simulink model "test_8m_0508"  (R2024a)
settings: Solver=FixedStepAuto  StartTime=0.0  StopTime=30  FixedStep=dt  RelTol=1e-3
values from neighbouring files (symbols this model uses):
  attitude_0 = [0; -90;  -0]    [ini_param_8m_0522.m]
  b = 4.0    (= 4)    [ini_param_8m_0522.m]
  cbar = 0.75    [ini_param_8m_0522.m]
  dt = 0.004    [ini_param_8m_0522.m]
  H = 1000    [ini_param_8m_0522.m]
  N_data = [0,200, 491, 804, 1077, 1344, 1559, 1832, 2078, 2318, 2579,            2864, 3117, 3371, 3608.2, 3872, 4055.7, 4291, 4507, 4739, 4935]'    [cal_motor.m]
  N_pwm = 0.01*[0, 5 ,10 ,15 ,20 ,25 ,30 ,35,40, 45 ,50 ,              55 ,60 ,65 ,70, 75, 80 , 85 ,90 ,95 ,100]'    [cal_motor.m]
  pitch_rate_K = 1    [ini_param_8m_0522.m]
  roll_rate_K = 1    [ini_param_8m_0522.m]
  S = 6.0    (= 6)    [ini_param_8m_0522.m]
  Ts = 0.05    [ini_param_8m_0522.m]
  Ts_sur = 0.25    [ini_param_8m_0522.m]
  yaw_rate_K = 1    [ini_param_8m_0522.m]
undefined symbols (not defined in the file or in its folder): sigbuilder_block, UAV
libraries: slpidlib x9, simulink_extras x6, sharedtransform x2, shared6dof x1
(part 1 of 11)
settings Model: Creator=elecl  LastModifiedBy=elecl

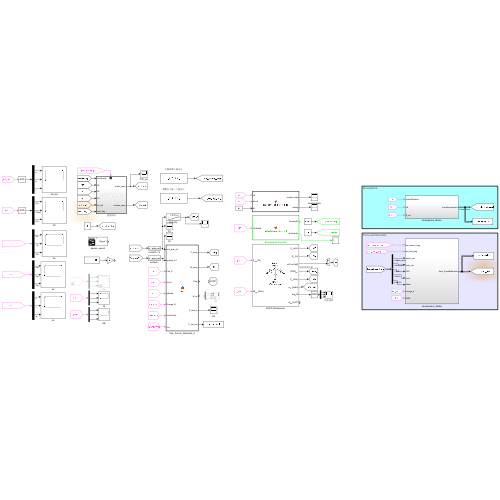
[thumbnail: Simulink's stored preview of the top-level diagram]
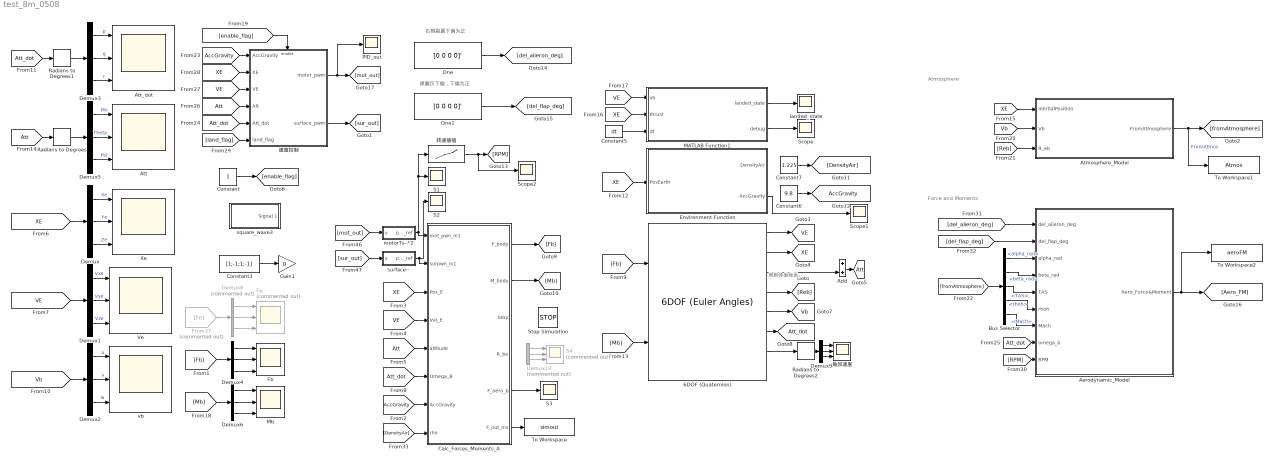
== system test_8m_0508 ==
  note: 地到体坐标系
  note: Force and Moments
  note: Atmosphere
  note: 右侧副翼下偏为正
  note: 襟翼仅下偏，下偏为正
  6DOF (Quaternion) : shared6dof/6DOF (Euler Angles)  units=Metric (MKS)  mtype=Fixed  rep=Quaternion  xme_0=[0 0 -H]  Vm_0=[1e-8 0 0]  eul_0=attitude_0*pi/180  pm_0=[0 0 0]  mass_0=StructAircraft.m  mass_e=0.5  mass_f=2.0  inertia=StructAircraft.inertia  inertia_e=eye(3)  inertia_f=2*eye(3)  k_quat=1.0  vre_flag=on  abi_flag=off  aMode=0  xme_statename=''  Vm_statename=''  eul_statename=''  quat_statename=''  pm_statename=''  mass_statename=''
  Add : Sum
  Aerodynamic_Model : Subsystem
  Atmosphere_Model : Subsystem
  Att : Scope  NumInputPorts=3
  Att_dot : Scope  NumInputPorts=3
  Bus Selector : BusSelector  OutputSignals=alpha_rad,beta_rad,TAS,rhoh,Mach
  Calc_Forces_Moments_A : MATLAB Function  TreatAsAtomicUnit=on  SystemSampleTime=0.004
  Constant : Constant
  Constant3 : Constant  Value=[1;-1;1;-1]
  Constant5 : Constant  Value=dt
  Constant6 : Constant  Value=9.8
  Constant7 : Constant  Value=1.225
  Demux{,1..6,9} (8 alike) : Demux  Outputs=3
  Demux10 : Demux  Commented=on  Outputs=3
  Demux8 : Demux  Commented=on  Outputs=3
  Environment Function : MATLAB Function  TreatAsAtomicUnit=on
  Fb : Scope  NumInputPorts=3
  Fe : Scope  Commented=on  NumInputPorts=3
  From37 : From  Commented=on  GotoTag=Fe
  Gain1 : Gain  Gain=0
  MATLAB Function1 : MATLAB Function  TreatAsAtomicUnit=on  SystemSampleTime=dt
  Mb : Scope  NumInputPorts=3
  One : Constant  Value=[0 0 0 0]'  OutDataTypeStr=Inherit: Inherit via back propagation
  One1 : Constant  Value=[0 0 0 0]'  OutDataTypeStr=Inherit: Inherit via back propagation
  PID_out : Scope
  Radians to Degrees : simulink_extras/Transformations/Radians to Degrees
  Radians to Degrees1 : simulink_extras/Transformations/Radians to Degrees
  Radians to Degrees2 : simulink_extras/Transformations/Radians to Degrees
  S1 : Scope
  S2 : Scope
  S3 : Scope
  S4 : Scope  Commented=on  NumInputPorts=3
  Scope : Scope
  Scope1 : Scope
  Scope2 : Scope
  Stop Simulation : Stop
  To Workspace : ToWorkspace  VariableName=simout  SaveFormat=Structure With Time  SampleTime=1
  To Workspace1 : ToWorkspace  VariableName=Atmos  SaveFormat=Structure  SampleTime=0.02
  To Workspace2 : ToWorkspace  VariableName=aeroFM  SaveFormat=Structure  SampleTime=0.02
  Ve : Scope  NumInputPorts=3
  Xe : Scope  NumInputPorts=3
  landed_state : Scope
  motorTs--*2 : Subsystem
  square_wave3 : Subsystem  Tag=STV Subsys  LoadFcn=sigbuilder_block('load');  StartFcn=sigbuilder_block('start');  StopFcn=sigbuilder_block('stop');  ClipboardFcn=sigbuilder_block('clipboard');  mask(Sigbuilder block){tuvar=[0:10]}
      mask help: Simulink:masks:SigbuilderBlock_MD
      mask init:
      | if ~strcmp(get_param(bdroot(gcbh),'SimulationStatus'),'stopped') tuvar = sigbuilder_block('maskInit'); end
      settings: CopyFcn=sigbuilder_block('copy');  DeleteFcn=sigbuilder_block('delete');  ModelCloseFcn=sigbuilder_block('modelClose');  PreSaveFcn=sigbuilder_block('preSave');  PauseFcn=sigbuilder_block('pause');  ContinueFcn=sigbuilder_block('continue');  NameChangeFcn=sigbuilder_block('namechange');  OpenFcn=sigbuilder_block('open',[239.25 91.5 550.5 408.75 ]);  CloseFcn=sigbuilder_block('close');
      mask Display: plot(0, 0, 100, 100,[2, 2, 32, 32, 2], [68, 8, 8, 68, 68],[32, 2], [38, 38], [32, 19, 2],[53, 60, 44], [32, 17, 17, 2],[16, 16, 31, 31]);txt = getActiveGroup(gcbh);text(2, 100, txt,'verticalAlignment', 'top');
  surface-- : Subsystem
  vb : Scope  NumInputPorts=3
  角加速度 : Scope  NumInputPorts=3
  转速插值 : Lookup_n-D  NumberOfTableDimensions=1  BreakpointsForDimension1=N_pwm  Table=N_data  InternalRulePriority=Speed  RndMeth=Simplest
  速度控制 : Subsystem  TreatAsAtomicUnit=on
  tag scope: AccGravity=global, Att=global, Att_dot=global, VE=global, Vb=global, XE=global
  wires:
  6DOF (Quaternion)/1 -> [VE]
  6DOF (Quaternion)/2 -> [XE]
  6DOF (Quaternion)/3 -> Add/2
  6DOF (Quaternion)/5 -> [Vb]
  6DOF (Quaternion)/6 -> [Att_dot]
  6DOF (Quaternion)/7 -> Radians to Degrees2/1
  Demux9/3 -> 角加速度/3
  Demux9/2 -> 角加速度/2
  Demux9/1 -> 角加速度/1
  Radians to Degrees2/1 -> Demux9/1
  [VE] -> Demux1/1
  Demux2/3 -> vb/3  "w"
  [Att_dot] -> Radians to Degrees1/1
  Demux2/1 -> vb/1  "u"
  Demux2/2 -> vb/2  "v"
  Demux5/1 -> Att/1  "Phi"
  Demux3/1 -> Att_dot/1  "p"
  Demux5/2 -> Att/2  "Theta"
  Demux3/3 -> Att_dot/3  "r"
  [Vb] -> Demux2/1
  Radians to Degrees/1 -> Demux5/1
  Demux3/2 -> Att_dot/2  "q"
  Demux5/3 -> Att/3  "Psi"
  [XE] -> Demux/1
  [Att] -> Radians to Degrees/1
  Demux/2 -> Xe/2  "Ye"
  Demux/3 -> Xe/3  "Ze"
  Demux1/3 -> Ve/3  "Vze"
  Demux1/2 -> Ve/2  "Vye"
  Demux/1 -> Xe/1  "Xe"
  Demux1/1 -> Ve/1  "Vxe"
  Environment Function/2(AccGravity) -> Scope1/1
  Constant7/1 -> [DensityAir]
  [XE] -> Environment Function/1(PosEarth)
  [XE] -> Calc_Forces_Moments_A/3(Pos_E)
  [VE] -> Calc_Forces_Moments_A/4(Vel_E)
  [Att] -> Calc_Forces_Moments_A/5(attitude)
  [Att_dot] -> Calc_Forces_Moments_A/6(Omega_B)
  Calc_Forces_Moments_A/2(M_body) -> [Mb]
  [Fb] -> 6DOF (Quaternion)/1
  [Mb] -> 6DOF (Quaternion)/2
  [Fb] -> Demux4/1
  Demux4/1 -> Fb/1
  Demux4/2 -> Fb/2
  Demux4/3 -> Fb/3
  Radians to Degrees1/1 -> Demux3/1
  [AccGravity] -> Calc_Forces_Moments_A/7(AccGravity)
  Demux6/3 -> Mb/3
  Demux6/2 -> Mb/2
  [Mb] -> Demux6/1
  Demux6/1 -> Mb/1
  速度控制/1(motor_pwm) -> PID_out/1, [mot_out]
  [enable_flag] -> 速度控制/Enable
  [AccGravity] -> 速度控制/1(AccGravity)
  [Att_dot] -> 速度控制/5(Att_dot)
  MATLAB Function1/1(landed_state) -> landed_state/1
  [VE] -> MATLAB Function1/1(vb)
  Constant5/1 -> MATLAB Function1/3(dt)
  [XE] -> MATLAB Function1/2(thrust)
  MATLAB Function1/2(debug) -> Scope/1
  [Att] -> 速度控制/4(Alt)
  [VE] -> 速度控制/3(VE)
  [XE] -> 速度控制/2(XE)
  Constant6/1 -> [AccGravity]
  [land_flag] -> 速度控制/6(land_flag)
  From37/1 -> Demux8/1
  Demux8/2 -> Fe/2
  Demux8/3 -> Fe/3
  Demux8/1 -> Fe/1
  Add/1 -> [Att]
  速度控制/2(surface_pwm) -> [sur_out]
  [sur_out] -> surface--/1(u)
  motorTs--*2/1(pwm_ref) -> 转速插值/1, S1/1, Calc_Forces_Moments_A/1(mot_pwn_in1)
  surface--/1(pwm_ref) -> S2/1, Calc_Forces_Moments_A/2(surpwn_in1)
  Constant/1 -> [enable_flag]
  [mot_out] -> motorTs--*2/1(u)
  Constant3/1 -> Gain1/1
  Demux10/1 -> S4/1
  Demux10/2 -> S4/2
  Demux10/3 -> S4/3
  Calc_Forces_Moments_A/1(F_body) -> [Fb]
  Calc_Forces_Moments_A/6(F_out_ms) -> To Workspace/1
  Aerodynamic_Model/1(Aero_Force&Moment) -> To Workspace2/1, [Aero_FM]
  Atmosphere_Model/1(FromAtmosphere) -> To Workspace1/1, [fromAtmosphere]  "FromAtmos"
  [XE] -> Atmosphere_Model/1(InertialPosition)
  [Vb] -> Atmosphere_Model/2(Vb)
  6DOF (Quaternion)/4 -> [Reb]
  [Reb] -> Atmosphere_Model/3(R_eb)
  Bus Selector/3 -> Aerodynamic_Model/5(TAS)  "<TAS>"
  Bus Selector/4 -> Aerodynamic_Model/6(rhoh)  "<rhoh>"
  Bus Selector/2 -> Aerodynamic_Model/4(beta_rad)  "<beta_rad>"
  [fromAtmosphere] -> Bus Selector/1
  Bus Selector/1 -> Aerodynamic_Model/3(alpha_rad)  "<alpha_rad>"
  Bus Selector/5 -> Aerodynamic_Model/7(Mach)  "<Mach>"
  [Att_dot] -> Aerodynamic_Model/8(omega_b)
  转速插值/1 -> Scope2/1, [RPM]
  [RPM] -> Aerodynamic_Model/9(RPM)
  One/1 -> [del_alieron_deg]
  One1/1 -> [del_flap_deg]
  [del_alieron_deg] -> Aerodynamic_Model/1(del_alieron_deg)
  [del_flap_deg] -> Aerodynamic_Model/2(del_flap_deg)
  [DensityAir] -> Calc_Forces_Moments_A/8(rho)
  Calc_Forces_Moments_A/5(F_aero_b) -> S3/1

== system test_8m_0508/Aerodynamic_Model ==
  del_alieron_deg : Inport
  del_flap_deg : Inport  Port=2
  alpha_rad : Inport  Port=3
  beta_rad : Inport  Port=4
  TAS : Inport  Port=5
  rhoh : Inport  Port=6
  Mach : Inport  Port=7
  omega_b : Inport  Port=8
  RPM : Inport  Port=9
  Absolute Force&Moment : Subsystem
  Bus Creator1 : BusCreator  Inputs=6
  Co-efficent Calculation in wing FoR : Subsystem
  Demux : Demux  Outputs=3
  Demux4 : Demux  Outputs=2
  Demux5 : Demux  Outputs=3
  Demux6 : Demux  Outputs=3
  Scope : Scope  NumInputPorts=6
  Scope1 : Scope  NumInputPorts=7
  Stability FoR to Body FoR : Subsystem
  Aero_Force&Moment : Outport
  wires:
  Demux/1 -> Co-efficent Calculation in wing FoR/3(p)  "p"
  omega_b/1 -> Demux/1
  [TAS] -> Co-efficent Calculation in wing FoR/8(TAS)
  TAS/1 -> [TAS]
  rhoh/1 -> [rhoh]
  Demux/2 -> Co-efficent Calculation in wing FoR/4(q)  "q"
  alpha_rad/1 -> Co-efficent Calculation in wing FoR/1(alpha_rad), Stability FoR to Body FoR/1(alpha_rad), Scope1/1
  del_alieron_deg/1 -> Co-efficent Calculation in wing FoR/6(del_alieron_deg)
  Demux/3 -> Co-efficent Calculation in wing FoR/5(r)  "r"
  beta_rad/1 -> Co-efficent Calculation in wing FoR/2(beta_rad)
  del_flap_deg/1 -> Co-efficent Calculation in wing FoR/7(del_flap_deg)
  Bus Creator1/1 -> Aero_Force&Moment/1
  Demux4/1 -> Demux5/1  "AeroForce_bFoR"
  Demux5/1 -> Scope/1, Bus Creator1/1  "X_Aero"
  Demux6/1 -> Scope/4, Bus Creator1/4  "L_Aero"
  Demux6/2 -> Scope/5, Bus Creator1/5  "M_aero"
  Demux5/2 -> Bus Creator1/2, Scope/2  "Y_Aero"
  Demux4/2 -> Demux6/1  "AeroMoment_b_AC"
  [rhoh] -> Absolute Force&Moment/1(rhoh)
  Stability FoR to Body FoR/2(AeroMoment_Coefficients_b_AC) -> Absolute Force&Moment/4(CM)  "AeroMoment_Coefficients_b_AC"
  Demux5/3 -> Scope/3, Bus Creator1/3  "Z_Aero"
  Stability FoR to Body FoR/1(AeroForce_Coefficients_bFoR) -> Absolute Force&Moment/3(CF)  "AeroForce_Coefficients_bFoR"
  Absolute Force&Moment/1(Aero_Force&Moment_ac) -> Demux4/1  "Aero_Force&Moment_ac"
  Demux6/3 -> Scope/6, Bus Creator1/6  "N_aero"
  [TAS] -> Absolute Force&Moment/2(TAS)
  Co-efficent Calculation in wing FoR/1(CL) -> Stability FoR to Body FoR/2(CL), Scope1/2  "CL"
  Co-efficent Calculation in wing FoR/2(CD) -> Scope1/3, Stability FoR to Body FoR/3(CD)  "CD"
  Co-efficent Calculation in wing FoR/3(CY) -> Scope1/4, Stability FoR to Body FoR/4(CY)  "CY"
  Co-efficent Calculation in wing FoR/4(Cl) -> Scope1/5, Stability FoR to Body FoR/5(Cl)  "Cl"
  Co-efficent Calculation in wing FoR/5(Cm) -> Scope1/6, Stability FoR to Body FoR/6(Cm)  "Cm"
  Co-efficent Calculation in wing FoR/6(Cn) -> Scope1/7, Stability FoR to Body FoR/7(Cn)  "Cn"
  Mach/1 -> [Mach]
  [Mach] -> Co-efficent Calculation in wing FoR/9(Mach)
  RPM/1 -> [RPM]
  [RPM] -> Co-efficent Calculation in wing FoR/10(RPM)

== system test_8m_0508/Atmosphere_Model ==
  InertialPosition : Inport
  Vb : Inport  Port=2
  R_eb : Inport  Port=3
  Bus Creator : BusCreator  Inputs=10
  Constant : Constant  Value=0
  Demux : Demux  Outputs=3
  EoM&Wind --> TAS : Subsystem
  Gain : Gain  Gain=-1
  ISA_upto20km : Subsystem
      mask Display: image('ISA_Temperature.png', [3,3,3,3,100,100]);
  Radians to Degrees : simulink_extras/Transformations/Radians to Degrees
  Scope : Scope
  TAS2CAS : Subsystem
      mask Display: image('TAS2CAS.png', [3,3,3,3,100,100]);
  Terminator : Terminator
  Terminator1 : Terminator
  FromAtmosphere : Outport
  wires:
  Demux/3 -> Gain/1
  Demux/2 -> Terminator1/1
  Demux/1 -> Terminator/1
  InertialPosition/1 -> Demux/1
  ISA_upto20km/4(ah) -> TAS2CAS/2(ah), Bus Creator/1  "ah"
  Gain/1 -> ISA_upto20km/1(h)
  Bus Creator/1 -> FromAtmosphere/1
  EoM&Wind --> TAS/4(aplhaDot_rps) -> Bus Creator/10  "alphaDot_rps"
  ISA_upto20km/2(Ph) -> Bus Creator/3, TAS2CAS/1(Ph)  "Ph"
  ISA_upto20km/1(Th) -> Bus Creator/2  "Th"
  TAS2CAS/1(Mach) -> Bus Creator/5  "Mach"
  EoM&Wind --> TAS/1(TAS) -> Bus Creator/7, TAS2CAS/3(TAS)  "TAS"
  EoM&Wind --> TAS/2(alpha_rad) -> Radians to Degrees/1, Bus Creator/8  "alpha_rad"
  EoM&Wind --> TAS/3(beta_rad) -> Bus Creator/9  "beta_rad"
  TAS2CAS/2(CAS) -> Bus Creator/6  "CAS"
  ISA_upto20km/3(rhoh) -> Bus Creator/4  "rhoh"
  Constant/1 -> EoM&Wind --> TAS/1(Wind_InertialX), EoM&Wind --> TAS/3(Wind_InertialZ), EoM&Wind --> TAS/2(Wind_InertialY)
  R_eb/1 -> EoM&Wind --> TAS/4(R_EB)
  Vb/1 -> EoM&Wind --> TAS/5(Vb)
  Radians to Degrees/1 -> Scope/1

== system test_8m_0508/motorTs--*2 ==
  u : Inport
  Demux5 : Demux  Outputs=8
  Mux5 : Mux  Inputs=8
  Transfer Fcn{,1..7} (8 alike) : TransferFcn  Denominator=[Ts 1]
  pwm_ref : Outport
  wires:
  Transfer Fcn7/1 -> Mux5/8
  Transfer Fcn6/1 -> Mux5/7
  Transfer Fcn5/1 -> Mux5/6
  Transfer Fcn4/1 -> Mux5/5
  Demux5/8 -> Transfer Fcn7/1
  Demux5/7 -> Transfer Fcn6/1
  Demux5/6 -> Transfer Fcn5/1
  Demux5/5 -> Transfer Fcn4/1
  Mux5/1 -> pwm_ref/1
  Transfer Fcn/1 -> Mux5/1
  u/1 -> Demux5/1
  Transfer Fcn1/1 -> Mux5/2
  Transfer Fcn3/1 -> Mux5/4
  Transfer Fcn2/1 -> Mux5/3
  Demux5/4 -> Transfer Fcn3/1
  Demux5/2 -> Transfer Fcn1/1
  Demux5/3 -> Transfer Fcn2/1
  Demux5/1 -> Transfer Fcn/1

== system test_8m_0508/square_wave3 ==
  Demux : Demux  Tag=STV Demux  Outputs=1
      settings: DisplayOption=none
  FromWs : FromWorkspace  Tag=STV FromWs  VariableName=tuvar
      SigBuilderData=|
      | common.afterFinalStr = 'Extrapolate'
      | common.sampleTime = 0
      | dataSet.timeRange = [0 80]
      | dataSet.name = 'Group 1'
      | sbobj.Groups.Name = 'Group 1'
      | sbobj.Groups.Signals.Name = 'Signal 1'
      | sbobj.Groups.Signals.XData = [0 5 5 36 80]
      | sbobj.Groups.Signals.YData = [0 0 1 1 1]
      | sbobj.Groups.TimeRange = [0 80]
  Signal 1 : Outport  Tag=STV Outport
  wires:
  FromWs/1 -> Demux/1
  Demux/1 -> Signal 1/1

== system test_8m_0508/surface-- ==
  u : Inport
  Demux5 : Demux  Outputs=8
  Mux5 : Mux  Inputs=8
  Transfer Fcn{,1..7} (8 alike) : TransferFcn  Denominator=[Ts_sur 1]
  pwm_ref : Outport
  wires:
  Demux5/1 -> Transfer Fcn/1
  Demux5/3 -> Transfer Fcn3/1
  Demux5/2 -> Transfer Fcn1/1
  Demux5/4 -> Transfer Fcn2/1
  Transfer Fcn3/1 -> Mux5/3
  Transfer Fcn2/1 -> Mux5/4
  Transfer Fcn1/1 -> Mux5/2
  u/1 -> Demux5/1
  Transfer Fcn/1 -> Mux5/1
  Mux5/1 -> pwm_ref/1
  Demux5/5 -> Transfer Fcn4/1
  Demux5/6 -> Transfer Fcn5/1
  Demux5/7 -> Transfer Fcn7/1
  Demux5/8 -> Transfer Fcn6/1
  Transfer Fcn6/1 -> Mux5/8
  Transfer Fcn4/1 -> Mux5/5
  Transfer Fcn5/1 -> Mux5/6
  Transfer Fcn7/1 -> Mux5/7

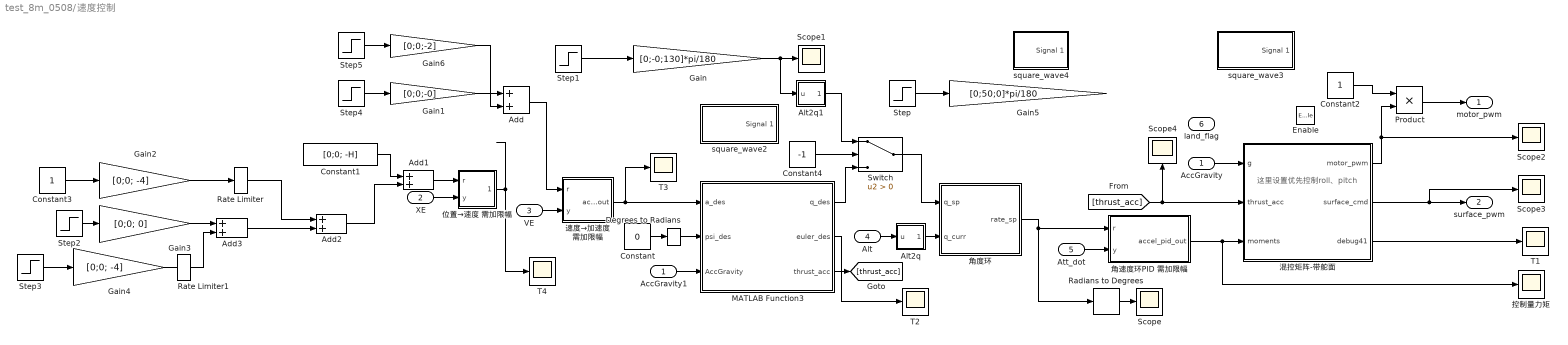
== system test_8m_0508/速度控制 ==
  note: 这里设置优先控制roll、pitch
  AccGravity : Inport
  XE : Inport  Port=2
  VE : Inport  Port=3
  Alt : Inport  Port=4
  Att_dot : Inport  Port=5
  land_flag : Inport  Port=6
  Enable : EnablePort
  AccGravity1 : InportShadow
  Add{,1..3} (4 alike) : Sum
  Alt2q : Subsystem
  Alt2q1 : Subsystem
  Constant : Constant  Value=0
  Constant1 : Constant  Value=[0;0; -H]
  Constant2 : Constant
  Constant3 : Constant
  Constant4 : Constant  Value=-1
  Degrees to Radians : simulink_extras/Transformations/Degrees to Radians
  Gain : Gain  Gain=[0;-0;130]*pi/180
  Gain1 : Gain  Gain=[0;0;-0]
  Gain2 : Gain  Gain=[0;0; -4]
  Gain3 : Gain  Gain=[0;0; 0]
  Gain4 : Gain  Gain=[0;0; -4]
  Gain5 : Gain  Gain=[0;50;0]*pi/180
  Gain6 : Gain  Gain=[0;0;-2]
  MATLAB Function3 : MATLAB Function  TreatAsAtomicUnit=on
  Product : Product
  Radians to Degrees : simulink_extras/Transformations/Radians to Degrees
  Rate Limiter : RateLimiter  RisingSlewLimit=5  FallingSlewLimit=-5  SampleTimeMode=inherited
  Rate Limiter1 : RateLimiter  RisingSlewLimit=5  FallingSlewLimit=-2  SampleTimeMode=inherited
  Scope{,1..4} (5 alike) : Scope
  Step : Step  Time=5  SampleTime=0
  Step1 : Step  Time=6  SampleTime=0
  Step2 : Step  Time=20  SampleTime=0
  Step3 : Step  Time=20  SampleTime=0
  Step4 : Step  Time=5  SampleTime=0
  Step5 : Step  Time=5  Before=1  After=0  SampleTime=0
  Switch : Switch  Criteria=u2 > Threshold  SaturateOnIntegerOverflow=off  InputSameDT=off
  T{1..4} (4 alike) : Scope
  square_wave2 : Subsystem  Tag=STV Subsys  LoadFcn=sigbuilder_block('load');  StartFcn=sigbuilder_block('start');  StopFcn=sigbuilder_block('stop');  ClipboardFcn=sigbuilder_block('clipboard');  mask(Sigbuilder block){tuvar=[0:10]}
      mask help: Simulink:masks:SigbuilderBlock_MD
      mask init:
      | if ~strcmp(get_param(bdroot(gcbh),'SimulationStatus'),'stopped') tuvar = sigbuilder_block('maskInit'); end
      settings: CopyFcn=sigbuilder_block('copy');  DeleteFcn=sigbuilder_block('delete');  ModelCloseFcn=sigbuilder_block('modelClose');  PreSaveFcn=sigbuilder_block('preSave');  PauseFcn=sigbuilder_block('pause');  ContinueFcn=sigbuilder_block('continue');  NameChangeFcn=sigbuilder_block('namechange');  OpenFcn=sigbuilder_block('open',[15 51 550.5 408.75 ]);  CloseFcn=sigbuilder_block('close');
      mask Display: plot(0, 0, 100, 100,[2, 2, 32, 32, 2], [68, 8, 8, 68, 68],[32, 2], [38, 38], [32, 19, 2],[53, 60, 44], [32, 17, 17, 2],[16, 16, 31, 31]);txt = getActiveGroup(gcbh);text(2, 100, txt,'verticalAlignment', 'top');
  square_wave3 : Subsystem  Tag=STV Subsys  LoadFcn=sigbuilder_block('load');  StartFcn=sigbuilder_block('start');  StopFcn=sigbuilder_block('stop');  ClipboardFcn=sigbuilder_block('clipboard');  mask(Sigbuilder block){tuvar=[0:10]}
      mask help: Simulink:masks:SigbuilderBlock_MD
      mask init:
      | if ~strcmp(get_param(bdroot(gcbh),'SimulationStatus'),'stopped') tuvar = sigbuilder_block('maskInit'); end
      settings: CopyFcn=sigbuilder_block('copy');  DeleteFcn=sigbuilder_block('delete');  ModelCloseFcn=sigbuilder_block('modelClose');  PreSaveFcn=sigbuilder_block('preSave');  PauseFcn=sigbuilder_block('pause');  ContinueFcn=sigbuilder_block('continue');  NameChangeFcn=sigbuilder_block('namechange');  OpenFcn=sigbuilder_block('open',[15 51 550.5 408.75 ]);  CloseFcn=sigbuilder_block('close');
      mask Display: plot(0, 0, 100, 100,[2, 2, 32, 32, 2], [68, 8, 8, 68, 68],[32, 2], [38, 38], [32, 19, 2],[53, 60, 44], [32, 17, 17, 2],[16, 16, 31, 31]);txt = getActiveGroup(gcbh);text(2, 100, txt,'verticalAlignment', 'top');
  square_wave4 : Subsystem  Tag=STV Subsys  LoadFcn=sigbuilder_block('load');  StartFcn=sigbuilder_block('start');  StopFcn=sigbuilder_block('stop');  ClipboardFcn=sigbuilder_block('clipboard');  mask(Sigbuilder block){tuvar=[0:10]}
      mask help: Simulink:masks:SigbuilderBlock_MD
      mask init:
      | if ~strcmp(get_param(bdroot(gcbh),'SimulationStatus'),'stopped') tuvar = sigbuilder_block('maskInit'); end
      settings: CopyFcn=sigbuilder_block('copy');  DeleteFcn=sigbuilder_block('delete');  ModelCloseFcn=sigbuilder_block('modelClose');  PreSaveFcn=sigbuilder_block('preSave');  PauseFcn=sigbuilder_block('pause');  ContinueFcn=sigbuilder_block('continue');  NameChangeFcn=sigbuilder_block('namechange');  OpenFcn=sigbuilder_block('open',[15 51 550.5 408.75 ]);  CloseFcn=sigbuilder_block('close');
      mask Display: plot(0, 0, 100, 100,[2, 2, 32, 32, 2], [68, 8, 8, 68, 68],[32, 2], [38, 38], [32, 19, 2],[53, 60, 44], [32, 17, 17, 2],[16, 16, 31, 31]);txt = getActiveGroup(gcbh);text(2, 100, txt,'verticalAlignment', 'top');
  位置→速度 需加限幅 : Subsystem
  控制量力矩 : Scope
  混控矩阵-带舵面 : MATLAB Function  TreatAsAtomicUnit=on
  角度环 : MATLAB Function  TreatAsAtomicUnit=on
  角速度环PID 需加限幅 : Subsystem
  速度→加速度 需加限幅 : Subsystem
  motor_pwm : Outport  InitialOutput=[0]
  surface_pwm : Outport  Port=2  InitialOutput=[0]
  wires:
  Att_dot/1 -> 角速度环PID 需加限幅/2(y)
  Step4/1 -> Gain1/1
  混控矩阵-带舵面/1(motor_pwm) -> Scope2/1, Product/2
  角速度环PID 需加限幅/1(accel_pid_out) -> 混控矩阵-带舵面/3(moments), 控制量力矩/1
  角度环/1(rate_sp) -> 角速度环PID 需加限幅/1(r), Radians to Degrees/1
  Alt2q/1(Quat) -> 角度环/2(q_curr)
  Alt/1 -> Alt2q/1(u)
  Gain/1 -> Alt2q1/1(u), Scope1/1
  AccGravity1/1 -> MATLAB Function3/3(AccGravity)
  Degrees to Radians/1 -> MATLAB Function3/2(psi_des)
  Alt2q1/1(Quat) -> Switch/1
  Radians to Degrees/1 -> Scope/1
  混控矩阵-带舵面/3(debug41) -> T1/1
  MATLAB Function3/3(thrust_acc) -> [thrust_acc]
  [thrust_acc] -> 混控矩阵-带舵面/2(thrust_acc), Scope4/1
  MATLAB Function3/2(euler_des) -> T2/1
  VE/1 -> 速度→加速度 需加限幅/2(y)
  Gain1/1 -> Add/1
  速度→加速度 需加限幅/1(accel_pid_out) -> MATLAB Function3/1(a_des), T3/1
  位置→速度 需加限幅/1(accel_pid_out) -> T4/1
  AccGravity/1 -> 混控矩阵-带舵面/1(g)
  MATLAB Function3/1(q_des) -> Switch/3
  Constant4/1 -> Switch/2
  Constant2/1 -> Product/1
  Product/1 -> motor_pwm/1
  Step/1 -> Gain5/1
  Switch/1 -> 角度环/1(q_sp)
  Step1/1 -> Gain/1
  Constant/1 -> Degrees to Radians/1
  XE/1 -> 位置→速度 需加限幅/2(y)
  Gain2/1 -> Rate Limiter/1
  Add1/1 -> 位置→速度 需加限幅/1(r)
  Constant1/1 -> Add1/1
  Constant3/1 -> Gain2/1
  Add2/1 -> Add1/2
  Add3/1 -> Add2/2
  Gain3/1 -> Add3/1
  Gain4/1 -> Add3/2
  Step2/1 -> Gain3/1
  Step3/1 -> Gain4/1
  Rate Limiter/1 -> Add2/1
  混控矩阵-带舵面/2(surface_cmd) -> surface_pwm/1, Scope3/1
  Add/1 -> 速度→加速度 需加限幅/1(r)
  Step5/1 -> Gain6/1
  Gain6/1 -> Add/2

== system test_8m_0508/Aerodynamic_Model/Absolute Force&Moment ==
  rhoh : Inport
  TAS : Inport  Port=2
  CF : Inport  Port=3
  CM : Inport  Port=4
  Constant : Constant  Value=b
  Constant1 : Constant  Value=cbar
  Demux1 : Demux  Outputs=3
  Demux2 : Demux  Outputs=3
  Mux : Mux  Inputs=6
  Product : Product
  Product1 : Product  Inputs=3
  Product2 : Product  Inputs=3
  Product3 : Product  Inputs=3
  Subsystem1 : Subsystem
  Aero_Force&Moment_ac : Outport
  wires:
  Demux2/3 -> Product3/2
  Demux1/3 -> Mux/3  "Z_aero"
  Constant1/1 -> Product2/3
  CF/1 -> Product/2
  CM/1 -> Demux2/1
  Demux1/1 -> Mux/1  "X_aero"
  Product3/1 -> Mux/6  "N_aero"
  Subsystem1/1(QS) -> [QS]  "QS"
  Constant/1 -> Product3/3, Product1/3
  Product/1 -> Demux1/1  "Aero_Forces"
  Demux2/1 -> Product1/2  "Cl"
  Demux2/2 -> Product2/2
  [QS] -> Product3/1, Product2/1, Product1/1
  Product2/1 -> Mux/5  "M_aero"
  Demux1/2 -> Mux/2  "Y_aero"
  Product1/1 -> Mux/4  "L_aero"
  rhoh/1 -> Subsystem1/1(rhoh)
  [QS] -> Product/1
  TAS/1 -> Subsystem1/2(TAS)
  Mux/1 -> Aero_Force&Moment_ac/1  "Aero_Force&Moment_ac"

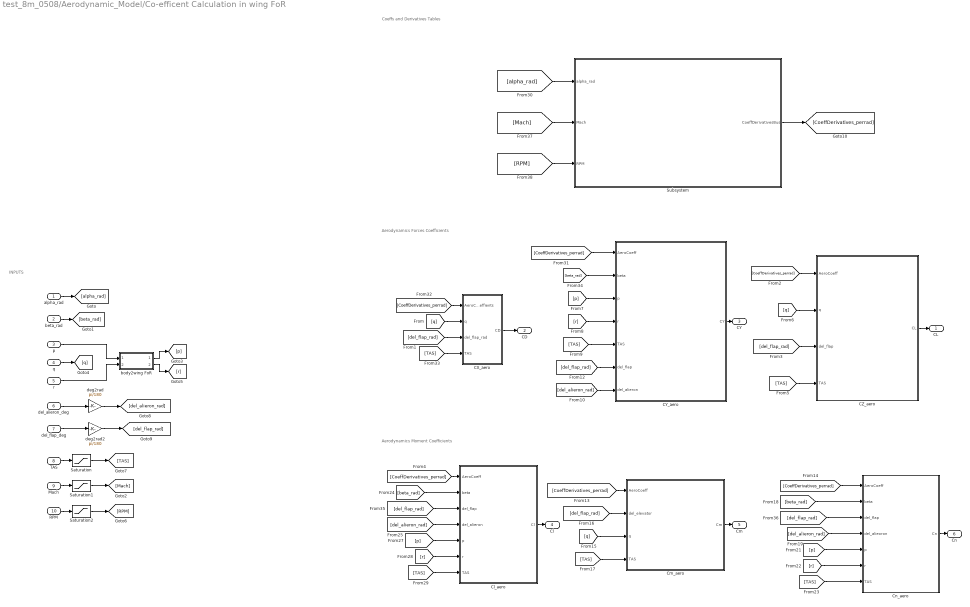
== system test_8m_0508/Aerodynamic_Model/Co-efficent Calculation in wing FoR ==
  note: Coeffs and Derivatives Tables
  note: INPUTS
  note: Aerodynamics Moment Coefficients
  note: Aerodynamics Forces Coefficients
  alpha_rad : Inport
  beta_rad : Inport  Port=2
  p : Inport  Port=3
  q : Inport  Port=4
  r : Inport  Port=5
  del_alieron_deg : Inport  Port=6
  del_flap_deg : Inport  Port=7
  TAS : Inport  Port=8
  Mach : Inport  Port=9
  RPM : Inport  Port=10
  CX_aero : Subsystem
  CY_aero : Subsystem
  CZ_aero : Subsystem
  Cl_aero : Subsystem
  Cm_aero : Subsystem
  Cn_aero : Subsystem
  Saturation : Saturate  UpperLimit=inf  LowerLimit=0.1
  Saturation1 : Saturate  UpperLimit=inf  LowerLimit=0
  Saturation2 : Saturate  UpperLimit=inf  LowerLimit=0
  Subsystem : Subsystem
  body2wing FoR : Subsystem
  deg2rad : Gain  Gain=pi/180
  deg2rad2 : Gain  Gain=pi/180
  CL : Outport
  CD : Outport  Port=2
  CY : Outport  Port=3
  Cl : Outport  Port=4
  Cm : Outport  Port=5
  Cn : Outport  Port=6
  wires:
  Saturation/1 -> [TAS]
  [del_flap_rad] -> CZ_aero/3(del_flap)
  alpha_rad/1 -> [alpha_rad]
  TAS/1 -> Saturation/1
  [r] -> Cn_aero/6(r)
  q/1 -> [q]
  beta_rad/1 -> [beta_rad]
  [r] -> Cl_aero/6(r)
  [q] -> Cm_aero/3(q)
  [del_flap_rad] -> CX_aero/3(del_flap_rad)
  [del_flap_rad] -> Cm_aero/2(del_elevator)
  Cm_aero/1(Cm) -> Cm/1
  [TAS] -> Cm_aero/4(TAS)
  [TAS] -> Cl_aero/7(TAS)
  [beta_rad] -> Cl_aero/2(beta)
  [p] -> Cl_aero/5(p)
  [beta_rad] -> Cn_aero/2(beta)
  [del_alieron_rad] -> Cl_aero/4(del_alieron)
  [TAS] -> CZ_aero/4(TAS)
  Cl_aero/1(Cl) -> Cl/1
  [del_alieron_rad] -> Cn_aero/4(del_alieoron)
  [p] -> Cn_aero/5(p)
  [TAS] -> Cn_aero/7(TAS)
  [q] -> CZ_aero/2(q)
  Cn_aero/1(Cn) -> Cn/1
  CX_aero/1(CD) -> CD/1
  CY_aero/1(CY) -> CY/1
  CZ_aero/1(CL) -> CL/1
  [CoeffDerivatives_perrad] -> CX_aero/1(AeroCoeffients)
  [TAS] -> CX_aero/4(TAS)
  [q] -> CX_aero/2(q)
  [CoeffDerivatives_perrad] -> CY_aero/1(AeroCoeff)
  [p] -> CY_aero/3(p)
  [r] -> CY_aero/4(r)
  [TAS] -> CY_aero/5(TAS)
  [del_alieron_rad] -> CY_aero/7(del_alieron)
  [del_flap_rad] -> CY_aero/6(del_flap)
  [beta_rad] -> CY_aero/2(beta)
  [CoeffDerivatives_perrad] -> CZ_aero/1(AeroCoeff)
  [CoeffDerivatives_perrad] -> Cl_aero/1(AeroCoeff)
  [CoeffDerivatives_perrad] -> Cm_aero/1(AeroCoeff)
  [CoeffDerivatives_perrad] -> Cn_aero/1(AeroCoeff)
  [del_flap_rad] -> Cl_aero/3(del_flap)
  [del_flap_rad] -> Cn_aero/3(del_flap)
  del_alieron_deg/1 -> deg2rad/1
  del_flap_deg/1 -> deg2rad2/1
  Mach/1 -> Saturation1/1
  Saturation1/1 -> [Mach]
  Saturation2/1 -> [RPM]
  RPM/1 -> Saturation2/1
  p/1 -> body2wing FoR/1(u_body)
  r/1 -> body2wing FoR/2(w_body)
  body2wing FoR/1(u_wing) -> [p]
  body2wing FoR/2(w_wing) -> [r]
  Subsystem/1(CoeffDerivativesBus) -> [CoeffDerivatives_perrad]
  [alpha_rad] -> Subsystem/1(alpha_rad)
  [Mach] -> Subsystem/2(Mach)
  [RPM] -> Subsystem/3(RPM)
  deg2rad/1 -> [del_alieron_rad]
  deg2rad2/1 -> [del_flap_rad]

== system test_8m_0508/Aerodynamic_Model/Stability FoR to Body FoR ==
  note: Cx = -CD
      | Cz = -CL
  note: In stability FoR
      | at AC
  note: In body FoR
      | at AC
  alpha_rad : Inport
  CL : Inport  Port=2
  CD : Inport  Port=3
  CY : Inport  Port=4
  Cl : Inport  Port=5
  Cm : Inport  Port=6
  Cn : Inport  Port=7
  Demux : Demux  Outputs=3
  Gain : Gain  Gain=-1
  Gain1 : Gain  Gain=-1
  Matrix Multiply : Product  Multiplication=Matrix(*)
  Matrix Multiply1 : Product  Multiplication=Matrix(*)
  Mux : Mux  Inputs=3
  Mux1 : Mux  Inputs=3
  Mux2 : Mux  Inputs=3
  StabilityToBody : Subsystem
  AeroForce_Coefficients_bFoR : Outport
  AeroMoment_Coefficients_b_AC : Outport  Port=2
  wires:
  Mux/1 -> Matrix Multiply/2  "AeroForce_Coefficients_sFoR"
  Cm/1 -> Mux1/2
  Mux1/1 -> Matrix Multiply1/2  "AeroMoment_Coefficients_sFoR"
  alpha_rad/1 -> StabilityToBody/1(AoA)
  Cn/1 -> Mux1/3
  Cl/1 -> Mux1/1
  Matrix Multiply1/1 -> AeroMoment_Coefficients_b_AC/1  "AeroMoment_Coefficients_b_AC"
  CD/1 -> Mux/1
  CY/1 -> Mux/2
  CL/1 -> Mux/3
  Matrix Multiply/1 -> Demux/1
  Demux/1 -> Gain/1
  Mux2/1 -> AeroForce_Coefficients_bFoR/1  "AeroForce_Coefficients_bFoR"
  Gain/1 -> Mux2/1
  Demux/2 -> Mux2/2
  Demux/3 -> Gain1/1
  Gain1/1 -> Mux2/3
  StabilityToBody/1(R_SB) -> Matrix Multiply1/1, Matrix Multiply/1

== system test_8m_0508/Atmosphere_Model/EoM&Wind --> TAS ==
  Wind_InertialX : Inport
  Wind_InertialY : Inport  Port=2
  Wind_InertialZ : Inport  Port=3
  R_EB : Inport  Port=4
  Vb : Inport  Port=5
  Add : Sum
  Asin : Trigonometry  Operator=asin
  Atan2 : Trigonometry  Operator=atan2
  Avoid_DivbyZero : Saturate  UpperLimit=inf  LowerLimit=0.1
  Demux1 : Demux  Outputs=3
  Derivative : Derivative
  Divide : Product  Inputs=*/
  Matrix Multiply : Product  Multiplication=Matrix(*)
  Mux : Mux  Inputs=3
  Sqrt : Sqrt
  Square : Math  Operator=square
  Square1 : Math  Operator=square
  Square2 : Math  Operator=square
  Sum : Sum  Inputs=+++
  body2wing FoR : Subsystem
  TAS : Outport
  alpha_rad : Outport  Port=2
  beta_rad : Outport  Port=3
  aplhaDot_rps : Outport  Port=4
  wires:
  Avoid_DivbyZero/1 -> Divide/2
  Divide/1 -> Asin/1
  Sum/1 -> Sqrt/1
  Wind_InertialX/1 -> Mux/1
  Demux1/1 -> body2wing FoR/1(u_body), Square/1  "u'"
  Demux1/3 -> body2wing FoR/2(w_body), Square2/1  "w'"
  Matrix Multiply/1 -> Add/1  "Wind_body"
  Atan2/1 -> alpha_rad/1, Derivative/1
  Sqrt/1 -> TAS/1, Avoid_DivbyZero/1
  Square/1 -> Sum/1
  Mux/1 -> Matrix Multiply/2
  Demux1/2 -> Divide/1, Square1/1  "v'"
  Square1/1 -> Sum/2
  Derivative/1 -> aplhaDot_rps/1
  Wind_InertialY/1 -> Mux/2
  Vb/1 -> Add/2
  Add/1 -> Demux1/1
  Asin/1 -> beta_rad/1
  R_EB/1 -> Matrix Multiply/1
  Wind_InertialZ/1 -> Mux/3
  Square2/1 -> Sum/3
  body2wing FoR/2(w_wing) -> Atan2/1
  body2wing FoR/1(u_wing) -> Atan2/2

== system test_8m_0508/Atmosphere_Model/ISA_upto20km ==
  h : Inport
  Constant1 : Constant  Value=101325
  Constant2 : Constant  Value=1.225
  Constant3 : Constant  Value=9.80665
  Constant4 : Constant  Value=287
  Subsystem : Subsystem
  Subsystem1 : Subsystem
  T0 : Constant  Value=288.16
  a : Constant  Value=-0.0065
  gamma : Constant  Value=1.4
  Th : Outport
  Ph : Outport  Port=2
  rhoh : Outport  Port=3
  ah : Outport  Port=4
  wires:
  gamma/1 -> [gamma]
  a/1 -> [a]
  Constant1/1 -> [P0]
  Constant4/1 -> [R]
  Constant2/1 -> [rho0]
  Constant3/1 -> [g0]
  h/1 -> [h]
  T0/1 -> [T0]
  [g0] -> Subsystem1/1(g0)
  [a] -> Subsystem1/2(a)
  [R] -> Subsystem1/3(R)
  [T0] -> Subsystem1/4(T0)
  [h] -> Subsystem1/5(h)
  [P0] -> Subsystem1/6(P0)
  [rho0] -> Subsystem1/7(rho0)
  Subsystem1/1(Th) -> Subsystem/1(Th), Th/1
  Subsystem1/2(Ph) -> Ph/1
  Subsystem1/3(rhoh) -> rhoh/1
  Subsystem/1(Speed of Sound at h) -> ah/1
  [gamma] -> Subsystem/2(gamma)
  [R] -> Subsystem/3(R)

== system test_8m_0508/Atmosphere_Model/TAS2CAS ==
  Ph : Inport
  ah : Inport  Port=2
  TAS : Inport  Port=3
  Add{,2..4,6..7} (6 alike) : Sum  Inputs=+-
  Add1 : Sum
  Add5 : Sum
  Constant{1,3..5,8..11} (8 alike) : Constant
  Constant2 : Constant  Value=2
  Constant6 : Constant  Value=101325
  Constant7 : Constant  Value=287
  Divide{,1..3} (4 alike) : Product  Inputs=*/
  Divide4 : Product  Inputs=/*
  Gain : Gain  Gain=2
  Power : Math  Operator=pow
  Power1 : Math  Operator=pow
  Product : Product
  Product1 : Product
  Product2 : Product
  Sqrt : Sqrt
  Square : Math  Operator=square
  Square1 : Math  Operator=square
  Subsystem : Subsystem
  Subsystem1 : Subsystem
  T0 : Constant  Value=288.16
  gamma : Constant  Value=1.4
  Mach : Outport
  CAS : Outport  Port=2
  wires:
  [gamma] -> Add6/1, Divide4/1
  [P0] -> Divide3/2
  Square1/1 -> Gain/1
  Product/1 -> Add1/1
  Constant3/1 -> Add1/2
  Add1/1 -> Power/1
  Constant2/1 -> Divide/2
  gamma/1 -> [gamma]
  Constant11/1 -> Add7/2
  Add/1 -> Divide/1
  Gain/1 -> Divide2/1
  Constant8/1 -> Add4/2
  Subsystem/1(Mach) -> Mach/1, Square/1
  Constant7/1 -> [R]
  [gamma] -> Add2/1, Divide1/1
  Constant6/1 -> [P0]
  Constant9/1 -> Add5/2
  Add7/1 -> Product2/1
  Divide4/1 -> Power1/2
  Add3/1 -> Product1/2
  Constant5/1 -> Add3/2
  Add4/1 -> Divide2/2
  Add2/1 -> Divide1/2
  Add5/1 -> Power1/1
  [gamma] -> Add/1
  Divide1/1 -> Power/2
  Divide3/1 -> Add5/1
  Subsystem1/1(a0) -> Square1/1
  Power1/1 -> Add7/1
  Constant1/1 -> Add/2
  Ph/1 -> Product1/1
  [gamma] -> Add4/1
  T0/1 -> [T0]
  [T0] -> Subsystem1/3(In3)
  Product1/1 -> Divide3/1  "Pt-Ps"
  TAS/1 -> Subsystem/2(TAS)
  [gamma] -> Subsystem1/1(In1)
  [R] -> Subsystem1/2(In2)
  Constant10/1 -> Add6/2
  Sqrt/1 -> CAS/1  "CAS"
  Add6/1 -> Divide4/2
  Power/1 -> Add3/1
  ah/1 -> Subsystem/1(ah)
  Divide/1 -> Product/2
  Constant4/1 -> Add2/2
  Square/1 -> Product/1
  Product2/1 -> Sqrt/1
  Divide2/1 -> Product2/2

== system test_8m_0508/速度控制/Alt2q ==
  u : Inport
  Rotation Angles to Quaternions : sharedtransform/Rotation Angles to Quaternions  rotationOrder=ZYX  aMode=aMode
  XYZ-ZYX : MATLAB Function  TreatAsAtomicUnit=on
  Quat : Outport
  wires:
  XYZ-ZYX/1(y) -> Rotation Angles to Quaternions/1
  u/1 -> XYZ-ZYX/1(u)
  Rotation Angles to Quaternions/1 -> Quat/1

== system test_8m_0508/速度控制/Alt2q1 ==
  u : Inport
  Rotation Angles to Quaternions : sharedtransform/Rotation Angles to Quaternions  rotationOrder=ZYX  aMode=aMode
  XYZ-ZYX : MATLAB Function  TreatAsAtomicUnit=on
  Quat : Outport
  wires:
  Rotation Angles to Quaternions/1 -> Quat/1
  u/1 -> XYZ-ZYX/1(u)
  XYZ-ZYX/1(y) -> Rotation Angles to Quaternions/1

== system test_8m_0508/速度控制/square_wave2 ==
  Demux : Demux  Tag=STV Demux  Outputs=1
      settings: DisplayOption=none
  FromWs : FromWorkspace  Tag=STV FromWs  VariableName=tuvar
      SigBuilderData=|
      | common.afterFinalStr = 'Extrapolate'
      | common.sampleTime = 0
      | dataSet.timeRange = [0 80]
      | dataSet.name = 'Group 1'
      | sbobj.Groups.Name = 'Group 1'
      | sbobj.Groups.Signals.Name = 'Signal 1'
      | sbobj.Groups.Signals.XData = [0 2 2 80]
      | sbobj.Groups.Signals.YData = [-1 -1 1 1]
      | sbobj.Groups.TimeRange = [0 80]
  Signal 1 : Outport  Tag=STV Outport
  wires:
  Demux/1 -> Signal 1/1
  FromWs/1 -> Demux/1

== system test_8m_0508/速度控制/square_wave3 ==
  Demux : Demux  Tag=STV Demux  Outputs=1
      settings: DisplayOption=none
  FromWs : FromWorkspace  Tag=STV FromWs  VariableName=tuvar
      SigBuilderData=|
      | common.afterFinalStr = 'Extrapolate'
      | common.sampleTime = 0
      | dataSet.timeRange = [0 80]
      | dataSet.name = 'Group 1'
      | sbobj.Groups.Name = 'Group 1'
      | sbobj.Groups.Signals.Name = 'Signal 1'
      | sbobj.Groups.Signals.XData = [0 35 36 80]
      | sbobj.Groups.Signals.YData = [1 1 0 0]
      | sbobj.Groups.TimeRange = [0 80]
  Signal 1 : Outport  Tag=STV Outport
  wires:
  FromWs/1 -> Demux/1
  Demux/1 -> Signal 1/1

== system test_8m_0508/速度控制/square_wave4 ==
  Demux : Demux  Tag=STV Demux  Outputs=1
      settings: DisplayOption=none
  FromWs : FromWorkspace  Tag=STV FromWs  VariableName=tuvar
      SigBuilderData=|
      | common.afterFinalStr = 'Extrapolate'
      | common.sampleTime = 0
      | dataSet.timeRange = [0 80]
      | dataSet.name = 'Group 1'
      | sbobj.Groups.Name = 'Group 1'
      | sbobj.Groups.Signals.Name = 'Signal 1'
      | sbobj.Groups.Signals.XData = [0 5 5 10 10 80]
      | sbobj.Groups.Signals.YData = [0 0 1 1 0 0]
      | sbobj.Groups.TimeRange = [0 80]
  Signal 1 : Outport  Tag=STV Outport
  wires:
  FromWs/1 -> Demux/1
  Demux/1 -> Signal 1/1

== system test_8m_0508/速度控制/位置→速度 需加限幅 ==
  r : Inport
  y : Inport  Port=2
  Add : Sum
  Constant : Constant  Value=[0;0;0]
  Demux1 : Demux  Outputs=3
  Demux2 : Demux  Outputs=3
  MATLAB Function : MATLAB Function  TreatAsAtomicUnit=on
  位置→速度 : slpidlib/PID Controller (2DOF)  Controller=PID  Form=Parallel  TimeDomain=Discrete-time  UseExternalTs=off  SampleTime=0.004  IntegratorMethod=Forward Euler  FilterMethod=Forward Euler  ControllerParametersSource=internal  P=UAV.pos_x.kp  I=UAV.pos_x.ki  UseKiTs=off  D=UAV.pos_x.kd  UseExternalDerivativeSource=off  N=100  UseFilter=on  b=1  c=0  TunerSelectOption=Transfer Function Based (PID Tuner App)  InitialConditionSource=internal  InitialConditionForIntegrator=0  InitialConditionForFilter=0  DifferentiatorICPrevScaledInput=0  ExternalReset=none  TrackingMode=off  Kt=1  LimitOutput=on  SatLimitsSource=internal  UpperSaturationLimit=UAV.pos_x.v_lim  LowerSaturationLimit=-UAV.pos_x.v_lim  LinearizeAsGain=on  AntiWindupMode=clamping  Kb=1  LimitIntegrator=off  UpperIntegratorSaturationLimit=inf  LowerIntegratorSaturationLimit=-inf  POutMin=[]  POutMax=[]  IOutMin=[]  IOutMax=[]  DOutMin=[]  DOutMax=[]  NOutMin=[]  NOutMax=[]  bOutMin=[]  bOutMax=[]  cOutMin=[]  cOutMax=[]  SumOutMin=[]  SumOutMax=[]  SaturationOutMin=[]  SaturationOutMax=[]  PParamMin=[]  PParamMax=[]  IParamMin=[]  IParamMax=[]  DParamMin=[]  DParamMax=[]  NParamMin=[]  NParamMax=[]  bParamMin=[]  bParamMax=[]  cParamMin=[]  cParamMax=[]  KbParamMin=[]  KbParamMax=[]  KtParamMin=[]  KtParamMax=[]  KbOutMin=[]  KbOutMax=[]  KtOutMin=[]  KtOutMax=[]  IntegratorOutMin=[]  IntegratorOutMax=[]  FilterOutMin=[]  FilterOutMax=[]  SumI1OutMin=[]  SumI1OutMax=[]  SumI2OutMin=[]  SumI2OutMax=[]  SumI3OutMin=[]  SumI3OutMax=[]  SumI4OutMin=[]  SumI4OutMax=[]  SumDOutMin=[]  SumDOutMax=[]  Sum1OutMin=[]  Sum1OutMax=[]  Sum2OutMin=[]  Sum2OutMax=[]  Sum3OutMin=[]  Sum3OutMax=[]  DifferentiatorOutMin=[]  DifferentiatorOutMax=[]  FilterDiffOutCoefMin=[]  FilterDiffOutCoefMax=[]  ReciprocalOutMin=[]  ReciprocalOutMax=[]  SumDenOutMin=[]  SumDenOutMax=[]  SumNumOutMin=[]  SumNumOutMax=[]  DivideOutMin=[]  DivideOutMax=[]  UdiffTsProdOutMin=[]  UdiffTsProdOutMax=[]  NTsProdOutMin=[]  NTsProdOutMax=[]  UintegralTsProdOutMin=[]  UintegralTsProdOutMax=[]  UngainTsProdOutMin=[]  UngainTsProdOutMax=[]  ClampingZeroOutDataTypeStr=Inherit: Inherit via back propagation  ClampingZeroOutMin=[]  ClampingZeroOutMax=[]  FilterDenConstantOutDataTypeStr=Inherit: Inherit via back propagation  FilterDenConstantOutMin=[]  FilterDenConstantOutMax=[]  PCopyOutDataTypeStr=Inherit: Inherit via back propagation  PCopyOutMin=[]  PCopyOutMax=[]  NCopyOutDataTypeStr=Inherit: Inherit via back propagation  NCopyOutMin=[]  NCopyOutMax=[]  IntegratorContinuousStateAttributes=''  IntegratorStateMustResolveToSignalObject=off  IntegratorRTWStateStorageClass=Auto  FilterContinuousStateAttributes=''  FilterStateMustResolveToSignalObject=off  FilterRTWStateStorageClass=Auto  ParallelPVariant=InternalParameters  IdealPVariant=Disabled  IVariant=InternalParameters  DVariant=InternalParameters  bVariant=InternalParameters  cVariant=InternalParameters  IntegratorVariant=Discrete  SatVariant=Enabled  AWVariant=DiscClampingParallel  PCopyVariant=Disabled  TRVariant=Disabled  FdbkBlocksVariant=Forward  IdealPFdbkVariant=Disabled  SatFdbkVariant=Disabled  DerivativeFilterVariant=ForwardEulerFilter  NVariant=InternalParameters  NCopyVariant=Disabled  FilterICVariant=InternalICsFilter  IntegratorICVariant=InternalICs  ExternalResetVariant=Disabled  TRSumVariant=Passthrough  SumFdbkVariant=Disabled  SumVariant=Sum_PID  TsampFilterVariant=InternalTs  TsampNgainVariant=Passthrough  TsampIntegralVariant=Disabled_SignalSpec  ExternalSaturationOutDataTypeStr=Inherit: Same as second input  DerivativeSourceVariant=ErrorSignal
  位置→速度1 : slpidlib/PID Controller (2DOF)  Controller=PID  Form=Parallel  TimeDomain=Discrete-time  UseExternalTs=off  SampleTime=0.004  IntegratorMethod=Forward Euler  FilterMethod=Forward Euler  ControllerParametersSource=internal  P=UAV.pos_y.kp  I=UAV.pos_y.ki  UseKiTs=off  D=UAV.pos_y.kd  UseExternalDerivativeSource=off  N=100  UseFilter=on  b=1  c=0  TunerSelectOption=Transfer Function Based (PID Tuner App)  InitialConditionSource=internal  InitialConditionForIntegrator=0  InitialConditionForFilter=0  DifferentiatorICPrevScaledInput=0  ExternalReset=none  TrackingMode=off  Kt=1  LimitOutput=on  SatLimitsSource=internal  UpperSaturationLimit=UAV.pos_y.v_lim  LowerSaturationLimit=-UAV.pos_y.v_lim  LinearizeAsGain=on  AntiWindupMode=clamping  Kb=1  LimitIntegrator=off  UpperIntegratorSaturationLimit=inf  LowerIntegratorSaturationLimit=-inf  POutMin=[]  POutMax=[]  IOutMin=[]  IOutMax=[]  DOutMin=[]  DOutMax=[]  NOutMin=[]  NOutMax=[]  bOutMin=[]  bOutMax=[]  cOutMin=[]  cOutMax=[]  SumOutMin=[]  SumOutMax=[]  SaturationOutMin=[]  SaturationOutMax=[]  PParamMin=[]  PParamMax=[]  IParamMin=[]  IParamMax=[]  DParamMin=[]  DParamMax=[]  NParamMin=[]  NParamMax=[]  bParamMin=[]  bParamMax=[]  cParamMin=[]  cParamMax=[]  KbParamMin=[]  KbParamMax=[]  KtParamMin=[]  KtParamMax=[]  KbOutMin=[]  KbOutMax=[]  KtOutMin=[]  KtOutMax=[]  IntegratorOutMin=[]  IntegratorOutMax=[]  FilterOutMin=[]  FilterOutMax=[]  SumI1OutMin=[]  SumI1OutMax=[]  SumI2OutMin=[]  SumI2OutMax=[]  SumI3OutMin=[]  SumI3OutMax=[]  SumI4OutMin=[]  SumI4OutMax=[]  SumDOutMin=[]  SumDOutMax=[]  Sum1OutMin=[]  Sum1OutMax=[]  Sum2OutMin=[]  Sum2OutMax=[]  Sum3OutMin=[]  Sum3OutMax=[]  DifferentiatorOutMin=[]  DifferentiatorOutMax=[]  FilterDiffOutCoefMin=[]  FilterDiffOutCoefMax=[]  ReciprocalOutMin=[]  ReciprocalOutMax=[]  SumDenOutMin=[]  SumDenOutMax=[]  SumNumOutMin=[]  SumNumOutMax=[]  DivideOutMin=[]  DivideOutMax=[]  UdiffTsProdOutMin=[]  UdiffTsProdOutMax=[]  NTsProdOutMin=[]  NTsProdOutMax=[]  UintegralTsProdOutMin=[]  UintegralTsProdOutMax=[]  UngainTsProdOutMin=[]  UngainTsProdOutMax=[]  ClampingZeroOutDataTypeStr=Inherit: Inherit via back propagation  ClampingZeroOutMin=[]  ClampingZeroOutMax=[]  FilterDenConstantOutDataTypeStr=Inherit: Inherit via back propagation  FilterDenConstantOutMin=[]  FilterDenConstantOutMax=[]  PCopyOutDataTypeStr=Inherit: Inherit via back propagation  PCopyOutMin=[]  PCopyOutMax=[]  NCopyOutDataTypeStr=Inherit: Inherit via back propagation  NCopyOutMin=[]  NCopyOutMax=[]  IntegratorContinuousStateAttributes=''  IntegratorStateMustResolveToSignalObject=off  IntegratorRTWStateStorageClass=Auto  FilterContinuousStateAttributes=''  FilterStateMustResolveToSignalObject=off  FilterRTWStateStorageClass=Auto  ParallelPVariant=InternalParameters  IdealPVariant=Disabled  IVariant=InternalParameters  DVariant=InternalParameters  bVariant=InternalParameters  cVariant=InternalParameters  IntegratorVariant=Discrete  SatVariant=Enabled  AWVariant=DiscClampingParallel  PCopyVariant=Disabled  TRVariant=Disabled  FdbkBlocksVariant=Forward  IdealPFdbkVariant=Disabled  SatFdbkVariant=Disabled  DerivativeFilterVariant=ForwardEulerFilter  NVariant=InternalParameters  NCopyVariant=Disabled  FilterICVariant=InternalICsFilter  IntegratorICVariant=InternalICs  ExternalResetVariant=Disabled  TRSumVariant=Passthrough  SumFdbkVariant=Disabled  SumVariant=Sum_PID  TsampFilterVariant=InternalTs  TsampNgainVariant=Passthrough  TsampIntegralVariant=Disabled_SignalSpec  ExternalSaturationOutDataTypeStr=Inherit: Same as second input  DerivativeSourceVariant=ErrorSignal
  位置→速度2 : slpidlib/PID Controller (2DOF)  Controller=PID  Form=Parallel  TimeDomain=Discrete-time  UseExternalTs=off  SampleTime=0.004  IntegratorMethod=Forward Euler  FilterMethod=Forward Euler  ControllerParametersSource=internal  P=UAV.pos_z.kp  I=UAV.pos_z.ki  UseKiTs=off  D=UAV.pos_z.kd  UseExternalDerivativeSource=off  N=100  UseFilter=on  b=1  c=0  TunerSelectOption=Transfer Function Based (PID Tuner App)  InitialConditionSource=internal  InitialConditionForIntegrator=0  InitialConditionForFilter=0  DifferentiatorICPrevScaledInput=0  ExternalReset=none  TrackingMode=off  Kt=1  LimitOutput=on  SatLimitsSource=internal  UpperSaturationLimit=UAV.pos_z.v_lim  LowerSaturationLimit=-UAV.pos_z.v_lim  LinearizeAsGain=on  AntiWindupMode=clamping  Kb=UAV.v2acc.kb_z  LimitIntegrator=off  UpperIntegratorSaturationLimit=inf  LowerIntegratorSaturationLimit=-inf  POutMin=[]  POutMax=[]  IOutMin=[]  IOutMax=[]  DOutMin=[]  DOutMax=[]  NOutMin=[]  NOutMax=[]  bOutMin=[]  bOutMax=[]  cOutMin=[]  cOutMax=[]  SumOutMin=[]  SumOutMax=[]  SaturationOutMin=[]  SaturationOutMax=[]  PParamMin=[]  PParamMax=[]  IParamMin=[]  IParamMax=[]  DParamMin=[]  DParamMax=[]  NParamMin=[]  NParamMax=[]  bParamMin=[]  bParamMax=[]  cParamMin=[]  cParamMax=[]  KbParamMin=[]  KbParamMax=[]  KtParamMin=[]  KtParamMax=[]  KbOutMin=[]  KbOutMax=[]  KtOutMin=[]  KtOutMax=[]  IntegratorOutMin=[]  IntegratorOutMax=[]  FilterOutMin=[]  FilterOutMax=[]  SumI1OutMin=[]  SumI1OutMax=[]  SumI2OutMin=[]  SumI2OutMax=[]  SumI3OutMin=[]  SumI3OutMax=[]  SumI4OutMin=[]  SumI4OutMax=[]  SumDOutMin=[]  SumDOutMax=[]  Sum1OutMin=[]  Sum1OutMax=[]  Sum2OutMin=[]  Sum2OutMax=[]  Sum3OutMin=[]  Sum3OutMax=[]  DifferentiatorOutMin=[]  DifferentiatorOutMax=[]  FilterDiffOutCoefMin=[]  FilterDiffOutCoefMax=[]  ReciprocalOutMin=[]  ReciprocalOutMax=[]  SumDenOutMin=[]  SumDenOutMax=[]  SumNumOutMin=[]  SumNumOutMax=[]  DivideOutMin=[]  DivideOutMax=[]  UdiffTsProdOutMin=[]  UdiffTsProdOutMax=[]  NTsProdOutMin=[]  NTsProdOutMax=[]  UintegralTsProdOutMin=[]  UintegralTsProdOutMax=[]  UngainTsProdOutMin=[]  UngainTsProdOutMax=[]  ClampingZeroOutDataTypeStr=Inherit: Inherit via back propagation  ClampingZeroOutMin=[]  ClampingZeroOutMax=[]  FilterDenConstantOutDataTypeStr=Inherit: Inherit via back propagation  FilterDenConstantOutMin=[]  FilterDenConstantOutMax=[]  PCopyOutDataTypeStr=Inherit: Inherit via back propagation  PCopyOutMin=[]  PCopyOutMax=[]  NCopyOutDataTypeStr=Inherit: Inherit via back propagation  NCopyOutMin=[]  NCopyOutMax=[]  IntegratorContinuousStateAttributes=''  IntegratorStateMustResolveToSignalObject=off  IntegratorRTWStateStorageClass=Auto  FilterContinuousStateAttributes=''  FilterStateMustResolveToSignalObject=off  FilterRTWStateStorageClass=Auto  ParallelPVariant=InternalParameters  IdealPVariant=Disabled  IVariant=InternalParameters  DVariant=InternalParameters  bVariant=InternalParameters  cVariant=InternalParameters  IntegratorVariant=Discrete  SatVariant=Enabled  AWVariant=DiscClampingParallel  PCopyVariant=Disabled  TRVariant=Disabled  FdbkBlocksVariant=Forward  IdealPFdbkVariant=Disabled  SatFdbkVariant=Disabled  DerivativeFilterVariant=ForwardEulerFilter  NVariant=InternalParameters  NCopyVariant=Disabled  FilterICVariant=InternalICsFilter  IntegratorICVariant=InternalICs  ExternalResetVariant=Disabled  TRSumVariant=Passthrough  SumFdbkVariant=Disabled  SumVariant=Sum_PID  TsampFilterVariant=InternalTs  TsampNgainVariant=Passthrough  TsampIntegralVariant=Disabled_SignalSpec  ExternalSaturationOutDataTypeStr=Inherit: Same as second input  DerivativeSourceVariant=ErrorSignal
  accel_pid_out : Outport
  wires:
  Demux1/3 -> 位置→速度2/1
  Add/1 -> accel_pid_out/1
  Constant/1 -> Add/2
  MATLAB Function/1(y) -> Add/1
  位置→速度/1 -> MATLAB Function/1(u1)
  位置→速度2/1 -> MATLAB Function/3(u3)
  Demux1/1 -> 位置→速度/1
  Demux2/3 -> 位置→速度2/2
  Demux2/2 -> 位置→速度1/2
  位置→速度1/1 -> MATLAB Function/2(u2)
  Demux1/2 -> 位置→速度1/1
  y/1 -> Demux2/1
  r/1 -> Demux1/1
  Demux2/1 -> 位置→速度/2
